simulink model "udpsend"  (Simulink 3.00)
settings: Solver=FixedStepDiscrete  StartTime=0.0  StopTime=inf  FixedStep=0.1  RelTol=1e-3
settings Model: ExtModeTrigMode=normal  ExtModeArmWhenConnect=on  LastModifiedBy=campa

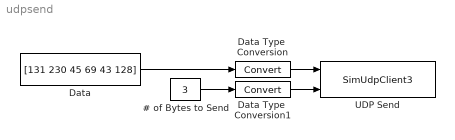
== system udpsend ==
  # of Bytes to Send : Constant  Value=3
  Data : Constant  Value=[131 230 45 69 43 128]
  Data Type  Conversion : DataTypeConversion  DataType=uint8  SaturateOnIntegerOverflow=on
  Data Type  Conversion1 : DataTypeConversion  DataType=uint32  SaturateOnIntegerOverflow=on
  UDP Send : S-Function  FunctionName=SimUdpClient3  Parameters=host,port,bufsize,T  PortCounts=[]  SFunctionModules=''  mask(UDP Send){host=127.0.0.1, port=64000, bufsize=6, T=0.1}
      mask prompts: host "Host name"; port "UDP Port"; bufsize "Buffer Size"; T "Sample Time"
      mask help:
      | This block sends bytes to an host computer via UDP/IP.
      |   The first input is the vector of data type uint8 (char) containing the
      |   bytes to be sent. The size of the vector is specified with the third
      |   parameter. The second input is a long integer containing the number
      |   of bytes to be sent from the first input vector (they could be less than
      |   the buffer size). The first parameter is either the hostname or the IP
      |   address of the host computer where the data need to be sent.
      |   The second parameter is the UDP port number.
      mask Help:
      | This block sends bytes to an host computer via UDP/IP.
      |   The first input is the vector of data type uint8 (char) containing the
      |   bytes to be sent. The size of the vector is specified with the third
      |   parameter. The second input is a long integer containing the number
      |   of bytes to be sent from the first input vector (they could be less than
      |   the buffer size). The first parameter is either the hostname or the IP
      |   address of the host computer where the data need to be sent.
      |   The second parameter is the UDP port number.
  wires:
  Data Type  Conversion/1 -> UDP Send/1
  Data/1 -> Data Type  Conversion/1
  # of Bytes to Send/1 -> Data Type  Conversion1/1
  Data Type  Conversion1/1 -> UDP Send/2
